simulink model "ESE4481_hw2"  (R2021a)
settings: Solver=VariableStepAuto  StartTime=0.0  StopTime=1  RelTol=1e-3
undefined symbols (not defined in the file or in its folder): coeffs, F_hover, g, J, J_inv, J_p, m, M_inv, omega_0, p_ned_0, Theta_0, theta_hover, V_b_0, Wrench_0, Wrench_step
libraries: vrlib x2
settings Model: Creator=tomwh  LastModifiedBy=tomwh
settings DataIOCC: ExternalInput=F_b,omega_bE,M_b

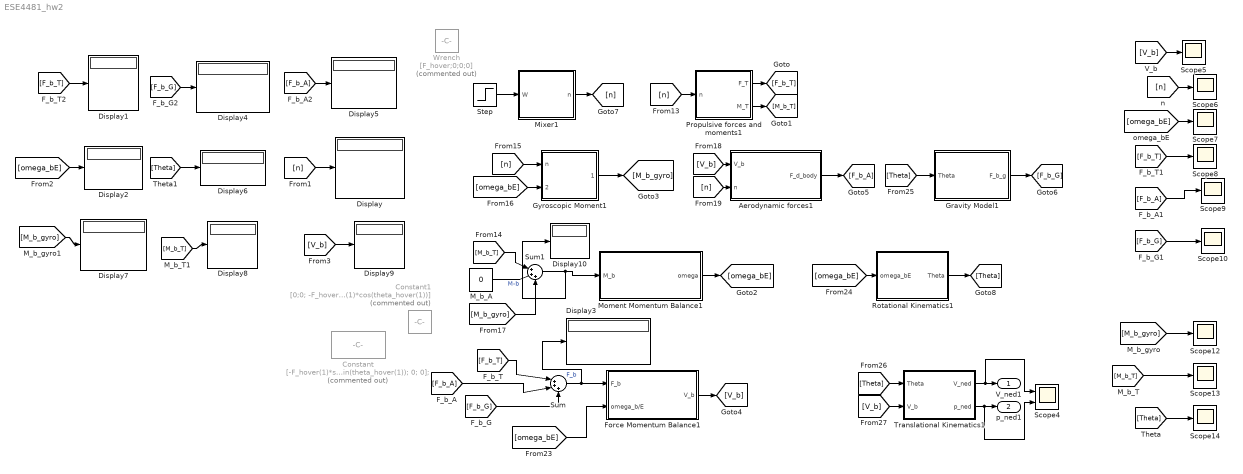
== system ESE4481_hw2 ==
  Aerodynamic forces1 : Subsystem
  Constant : Constant  Commented=on  Value=[-F_hover(1)*sin(theta_hover(1)); 0; 0];
  Constant1 : Constant  Commented=on  Value=[0;0; -F_hover(1)*cos(theta_hover(1))]
  Display{,1..10} (11 alike) : Display
  Force Momentum Balance1 : Subsystem
  Gravity Model1 : Subsystem
  Gyroscopic Moment1 : Subsystem
  M_b_A : Constant  Value=0
  Mixer1 : Subsystem
  Moment Momentum Balance1 : Subsystem
  Propulsive forces and moments1 : Subsystem
  Rotational Kinematics1 : Subsystem
  Scope{5..10,12..14} (9 alike) : Scope
  Scope4 : Scope  NumInputPorts=2
  Step : Step  Time=0.4  Before=Wrench_0  After=Wrench_step  SampleTime=0
  Sum : Sum  Inputs=|+++
  Sum1 : Sum  Inputs=|+++
  Translational Kinematics1 : Subsystem
  Wrench : Constant  Commented=on  Value=[F_hover;0;0;0]
  V_ned1 : Outport
  p_ned1 : Outport  Port=2
  wires:
  Mixer1/1(n) -> [n]
  [n] -> Propulsive forces and moments1/1(n)
  Propulsive forces and moments1/1(F_T) -> [F_b_T]
  Propulsive forces and moments1/2(M_T) -> [M_b_T]
  [M_b_T] -> Sum1/1
  M_b_A/1 -> Sum1/2
  [n] -> Gyroscopic Moment1/1(n)
  Moment Momentum Balance1/1(omega) -> [omega_bE]
  [omega_bE] -> Gyroscopic Moment1/2(omega_bE)
  Gyroscopic Moment1/1(M_gyro) -> [M_b_gyro]
  Sum1/1 -> Display10/1, Moment Momentum Balance1/1(M_b)  "M-b"
  [M_b_gyro] -> Sum1/3
  Force Momentum Balance1/1(V_b) -> [V_b]
  [V_b] -> Aerodynamic forces1/1(V_b)
  [n] -> Aerodynamic forces1/2(n)
  Aerodynamic forces1/1(F_d_body) -> [F_b_A]
  Gravity Model1/1(F_b_g) -> [F_b_G]
  [F_b_G] -> Sum/3
  Sum/1 -> Display3/1, Force Momentum Balance1/1(F_b)  "F_b"
  [omega_bE] -> Force Momentum Balance1/2(omega_b/E)
  [omega_bE] -> Rotational Kinematics1/1(omega_bE)
  Rotational Kinematics1/1(Theta) -> [Theta]
  [Theta] -> Gravity Model1/1(Theta)
  [Theta] -> Translational Kinematics1/1(Theta)
  [V_b] -> Translational Kinematics1/2(V_b)
  Translational Kinematics1/2(p_ned) -> Scope4/2, p_ned1/1
  Translational Kinematics1/1(V_ned) -> Scope4/1, V_ned1/1
  [V_b] -> Scope5/1
  [n] -> Scope6/1
  [omega_bE] -> Scope7/1
  [F_b_T] -> Scope8/1
  [Theta] -> Scope14/1
  [M_b_T] -> Scope13/1
  [M_b_gyro] -> Scope12/1
  [F_b_G] -> Scope10/1
  [F_b_A] -> Scope9/1
  [F_b_T] -> Sum/1
  [F_b_A] -> Sum/2
  [n] -> Display/1
  [F_b_T] -> Display1/1
  [omega_bE] -> Display2/1
  [F_b_G] -> Display4/1
  [F_b_A] -> Display5/1
  [Theta] -> Display6/1
  [M_b_gyro] -> Display7/1
  [M_b_T] -> Display8/1
  [V_b] -> Display9/1
  Step/1 -> Mixer1/1(W)

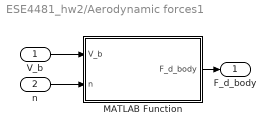
== system ESE4481_hw2/Aerodynamic forces1 ==
  V_b : Inport
  n : Inport  Port=2
  MATLAB Function : MATLAB Function  TreatAsAtomicUnit=on
  F_d_body : Outport
  wires:
  MATLAB Function/1(F_d_body) -> F_d_body/1
  n/1 -> MATLAB Function/2(n)
  V_b/1 -> MATLAB Function/1(V_b)

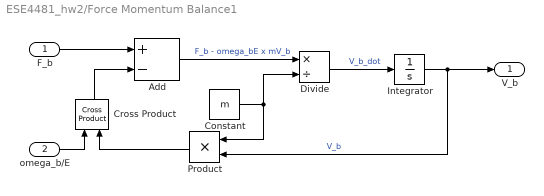
== system ESE4481_hw2/Force Momentum Balance1 ==
  F_b : Inport
  omega_b/E : Inport  Port=2
  Add : Sum  Inputs=+-
  Constant : Constant  Value=m
  Cross Product : vrlib/Utilities/Cross Product
  Divide : Product  Inputs=*/
  Integrator : Integrator  InitialCondition=V_b_0
      settings: AttributesFormatString=%<InitialCondition>
  Product : Product
  V_b : Outport
  wires:
  omega_b/E/1 -> Cross Product/1
  F_b/1 -> Add/1
  Integrator/1 -> V_b/1, Product/2  "V_b"
  Constant/1 -> Divide/2, Product/1
  Divide/1 -> Integrator/1  "V_b_dot"
  Add/1 -> Divide/1  "F_b - omega_bE x mV_b"
  Cross Product/1 -> Add/2
  Product/1 -> Cross Product/2

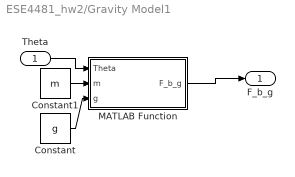
== system ESE4481_hw2/Gravity Model1 ==
  Theta : Inport
  Constant : Constant  Value=g
  Constant1 : Constant  Value=m
  MATLAB Function : MATLAB Function  TreatAsAtomicUnit=on
  F_b_g : Outport
  wires:
  Theta/1 -> MATLAB Function/1(Theta)
  MATLAB Function/1(F_b_g) -> F_b_g/1
  Constant/1 -> MATLAB Function/3(g)
  Constant1/1 -> MATLAB Function/2(m)

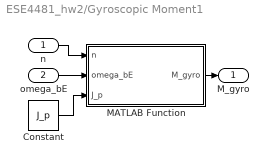
== system ESE4481_hw2/Gyroscopic Moment1 ==
  n : Inport
  omega_bE : Inport  Port=2
  Constant : Constant  Value=J_p
  MATLAB Function : MATLAB Function  TreatAsAtomicUnit=on
  M_gyro : Outport
  wires:
  n/1 -> MATLAB Function/1(n)
  MATLAB Function/1(M_gyro) -> M_gyro/1
  omega_bE/1 -> MATLAB Function/2(omega_bE)
  Constant/1 -> MATLAB Function/3(J_p)

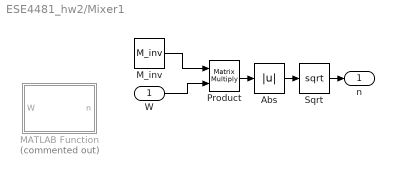
== system ESE4481_hw2/Mixer1 ==
  W : Inport
  Abs : Abs
  MATLAB Function : MATLAB Function  Commented=on  TreatAsAtomicUnit=on
  M_inv : Constant  Value=M_inv
  Product : Product  Multiplication=Matrix(*)
  Sqrt : Sqrt  SaturateOnIntegerOverflow=on
  n : Outport
  wires:
  M_inv/1 -> Product/1
  W/1 -> Product/2
  Product/1 -> Abs/1
  Abs/1 -> Sqrt/1
  Sqrt/1 -> n/1

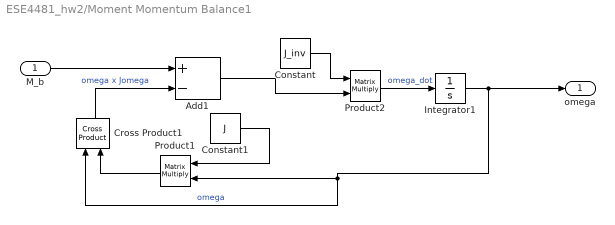
== system ESE4481_hw2/Moment Momentum Balance1 ==
  M_b : Inport
  Add1 : Sum  Inputs=+-
  Constant : Constant  Value=J_inv
  Constant1 : Constant  Value=J
  Cross Product1 : vrlib/Utilities/Cross Product
  Integrator1 : Integrator  InitialCondition=omega_0
      settings: AttributesFormatString=%<InitialCondition>
  Product1 : Product  Multiplication=Matrix(*)
  Product2 : Product  Multiplication=Matrix(*)
  omega : Outport
  wires:
  Constant1/1 -> Product1/1
  Cross Product1/1 -> Add1/2  "omega x Jomega"
  Integrator1/1 -> omega/1, Cross Product1/1, Product1/2  "omega"
  Product1/1 -> Cross Product1/2
  Product2/1 -> Integrator1/1  "omega_dot"
  M_b/1 -> Add1/1
  Constant/1 -> Product2/1
  Add1/1 -> Product2/2

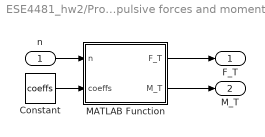
== system ESE4481_hw2/Propulsive forces and moments1 ==
  n : Inport
  Constant : Constant  Value=coeffs
  MATLAB Function : MATLAB Function  TreatAsAtomicUnit=on
  F_T : Outport
  M_T : Outport  Port=2
  wires:
  MATLAB Function/2(M_T) -> M_T/1
  n/1 -> MATLAB Function/1(n)
  MATLAB Function/1(F_T) -> F_T/1
  Constant/1 -> MATLAB Function/2(coeffs)

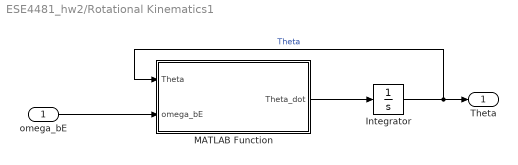
== system ESE4481_hw2/Rotational Kinematics1 ==
  omega_bE : Inport
  Integrator : Integrator  InitialCondition=Theta_0
      settings: AttributesFormatString=%<InitialCondition>
  MATLAB Function : MATLAB Function  TreatAsAtomicUnit=on
  Theta : Outport
  wires:
  Integrator/1 -> MATLAB Function/1(Theta), Theta/1  "Theta"
  omega_bE/1 -> MATLAB Function/2(omega_bE)
  MATLAB Function/1(Theta_dot) -> Integrator/1

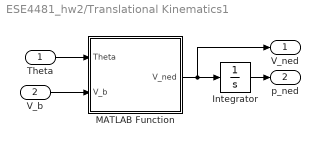
== system ESE4481_hw2/Translational Kinematics1 ==
  Theta : Inport
  V_b : Inport  Port=2
  Integrator : Integrator  InitialCondition=p_ned_0
      settings: AttributesFormatString=%<InitialCondition>
  MATLAB Function : MATLAB Function  TreatAsAtomicUnit=on
  V_ned : Outport
  p_ned : Outport  Port=2
  wires:
  MATLAB Function/1(V_ned) -> V_ned/1, Integrator/1
  V_b/1 -> MATLAB Function/2(V_b)
  Integrator/1 -> p_ned/1
  Theta/1 -> MATLAB Function/1(Theta)

== matlab function ESE4481_hw2/Propulsive forces and moments1/MATLAB Function ==
  data: n input; F_T output; M_T output; coeffs input
function [F_T,M_T]= fcn(n,coeffs)
a = coeffs(1);
b = coeffs(2);
c = coeffs(3);
d = coeffs(4);
F_T = [0;0; -a*(n(1)^2 + n(2)^2 + n(3)^2 + n(4)^2)];
M_T = [b*(n(1)^2 - n(2)^2 - n(3)^2 + n(4)^2); c*(n(1)^2 + n(2)^2 - n(3)^2 - n(4)^2); d*(-n(1)^2 + n(2)^2 - n(3)^2 + n(4)^2)];

== matlab function ESE4481_hw2/Aerodynamic forces1/MATLAB Function ==
  data: V_b input; F_d_body output; n input
function F_d_body = fcn(V_b,n)
rho = 1.293;
D = 0.066;
C_t = @(n) 4.375*10^(-5)*n + 0.0704;
K_c = 0.22;
K = [K_c 0 0;
     0 K_c 0;
     0 0 0];
F_d_body = -rho*C_t(abs(n(2)))*D^4*(n(1)^2 + n(2)^2 + n(3)^2 + n(4)^2)*K*V_b;

== matlab function ESE4481_hw2/Gyroscopic Moment1/MATLAB Function ==
  data: n input; M_gyro output; omega_bE input; J_p input
function M_gyro = fcn(n,omega_bE,J_p)
    H = [0;0; J_p*2*pi*(n(1)-n(2)+n(3)-n(4))];
M_gyro = cross(omega_bE,H);

== matlab function ESE4481_hw2/Gravity Model1/MATLAB Function ==
  data: Theta input; F_b_g output; m input; g input
function F_b_g = fcn(Theta,m,g)
phi = Theta(1);
theta = Theta(2);
psi = Theta(3);
R_phi = [1 0 0;
         0 cos(phi) sin(phi);
         0 -sin(phi) cos(phi)];
R_theta = [cos(theta) 0 -sin(theta);
           0 1 0;
           sin(theta) 0 cos(theta)];
R_psi = [cos(psi) sin(psi) 0;
         -sin(psi) cos(psi) 0;
         0 0 1];
R_b_E = R_phi*R_theta*R_psi;
F_b_g = R_b_E*[0; 0; m*g];

== matlab function ESE4481_hw2/Rotational Kinematics1/MATLAB Function ==
  data: Theta input; Theta_dot output; omega_bE input
function Theta_dot = fcn(Theta,omega_bE)
    phi = Theta(1);
    theta = Theta(2);
    H_inv = [1 sin(phi)*tan(theta) cos(phi)*tan(theta);
             0 cos(phi) -sin(phi);
             0 sin(phi)*sec(theta) cos(phi)*sec(theta)];
Theta_dot = H_inv*omega_bE;

== matlab function ESE4481_hw2/Translational Kinematics1/MATLAB Function ==
  data: Theta input; V_ned output; V_b input
function V_ned = fcn(Theta,V_b)
phi = Theta(1);
theta = Theta(2);
psi = Theta(3);
R_phi = [1 0 0;
         0 cos(phi) sin(phi);
         0 -sin(phi) cos(phi)];
R_theta = [cos(theta) 0 -sin(theta);
           0 1 0;
           sin(theta) 0 cos(theta)];
R_psi = [cos(psi) sin(psi) 0;
         -sin(psi) cos(psi) 0;
         0 0 1];
R = R_phi*R_theta*R_psi;
% R = [cos(psi)*cos(theta) cos(theta)*sin(psi) -sin(theta);
%      cos(psi)*sin(phi)*sin(theta)-cos(phi)*sin(psi) cos(phi)*cos(psi)+sin(phi)*sin(psi)*sin(theta) cos(theta)*sin(phi)
%      sin(phi)*sin(psi)+cos(phi)*cos(psi)*sin(theta) cos(phi)*sin(psi)*sin(theta)-cos(psi)*sin(phi) cos(phi)*cos(theta)];
V_ned = R\V_b;

== matlab function ESE4481_hw2/Mixer1/MATLAB Function ==
  data: W input; n output
function n = getMotorSpeeds(W)
% a = 2.034763500512882e-06;
% b = 9.690561171192599e-08;
% c = b;
% d = 1.056628184682481e-08;
rho = 1.293;
D = 0.066;
C_t = @(n) 4.375*10^(-5)*n + 0.0704; 
C_p = 0.041;
dist_xy = 0.047625; 
n_eq = 2.893014369037372e+02;
a = C_t(n_eq)*rho*D^4;
b = C_t(n_eq)*rho*D^4*dist_xy;
c = b;
d = C_p*rho*D^5/(2*pi);
M = [a a a a;
    b -b -b b;
    c c -c -c;
    -d d -d d];
nu = abs(M\W);
n = sqrt(nu);
